simulink model "c00007M_harness"  (R2018a)
settings: Solver=FixedStepAuto  StartTime=0.0  StopTime=300  FixedStep=0.1  RelTol=1e-3
undefined symbols (not defined in the file): A1, hmax, R1, R2, sigbuilder_block, TempThreshold
(part 4 of 14)

== system c00007M_harness/M014/Tank1 ==
  CT1 : Inport
  F1 : Inport  Port=2
  E1 : Inport  Port=3
  MR1 : Inport  Port=4
  T1 : Inport  Port=5
  EB1 : Inport  Port=6
  Control : Subsystem
  Memory : Memory
  TankModel : Subsystem
  LL1 : Outport
  wires:
  TankModel/1(LiquidLevel) -> Memory/1, LL1/1
  Control/2(LiquidOut) -> TankModel/2(LiquidOut)
  Memory/1 -> Control/8(LiquidLevel)
  MR1/1 -> Control/3(ManualReference)
  CT1/1 -> Control/2(StartMaintenance), Control/1(ControlType)
  F1/1 -> Control/4(Fill)
  E1/1 -> Control/5(Empty)
  EB1/1 -> Control/6(EmergencyButton)
  T1/1 -> Control/7(Temperature)
  Control/1(LiquidIn) -> TankModel/1(LiquidIn)

== system c00007M_harness/M015/Tank1 ==
  CT1 : Inport
  F1 : Inport  Port=2
  E1 : Inport  Port=3
  MR1 : Inport  Port=4
  T1 : Inport  Port=5
  EB1 : Inport  Port=6
  Control : Subsystem
  Memory : Memory
  TankModel : Subsystem
  LL1 : Outport
  wires:
  TankModel/1(LiquidLevel) -> Memory/1, LL1/1
  Control/2(LiquidOut) -> TankModel/2(LiquidOut)
  Memory/1 -> Control/8(LiquidLevel)
  MR1/1 -> Control/3(ManualReference)
  CT1/1 -> Control/2(StartMaintenance), Control/1(ControlType)
  F1/1 -> Control/4(Fill)
  E1/1 -> Control/5(Empty)
  EB1/1 -> Control/6(EmergencyButton)
  T1/1 -> Control/7(Temperature)
  Control/1(LiquidIn) -> TankModel/1(LiquidIn)

== system c00007M_harness/M016/Tank1 ==
  CT1 : Inport
  F1 : Inport  Port=2
  E1 : Inport  Port=3
  MR1 : Inport  Port=4
  T1 : Inport  Port=5
  EB1 : Inport  Port=6
  Control : Subsystem
  Memory : Memory
  TankModel : Subsystem
  LL1 : Outport
  wires:
  TankModel/1(LiquidLevel) -> Memory/1, LL1/1
  Control/2(LiquidOut) -> TankModel/2(LiquidOut)
  Memory/1 -> Control/8(LiquidLevel)
  MR1/1 -> Control/3(ManualReference)
  CT1/1 -> Control/2(StartMaintenance), Control/1(ControlType)
  F1/1 -> Control/4(Fill)
  E1/1 -> Control/5(Empty)
  EB1/1 -> Control/6(EmergencyButton)
  T1/1 -> Control/7(Temperature)
  Control/1(LiquidIn) -> TankModel/1(LiquidIn)

== system c00007M_harness/M017/Tank1 ==
  CT1 : Inport
  F1 : Inport  Port=2
  E1 : Inport  Port=3
  MR1 : Inport  Port=4
  T1 : Inport  Port=5
  EB1 : Inport  Port=6
  Control : Subsystem
  Memory : Memory
  TankModel : Subsystem
  LL1 : Outport
  wires:
  TankModel/1(LiquidLevel) -> Memory/1, LL1/1
  Control/2(LiquidOut) -> TankModel/2(LiquidOut)
  Memory/1 -> Control/8(LiquidLevel)
  MR1/1 -> Control/3(ManualReference)
  CT1/1 -> Control/2(StartMaintenance), Control/1(ControlType)
  F1/1 -> Control/4(Fill)
  E1/1 -> Control/5(Empty)
  EB1/1 -> Control/6(EmergencyButton)
  T1/1 -> Control/7(Temperature)
  Control/1(LiquidIn) -> TankModel/1(LiquidIn)

== system c00007M_harness/M018/Tank1 ==
  CT1 : Inport
  F1 : Inport  Port=2
  E1 : Inport  Port=3
  MR1 : Inport  Port=4
  T1 : Inport  Port=5
  EB1 : Inport  Port=6
  Control : Subsystem
  Memory : Memory
  TankModel : Subsystem
  LL1 : Outport
  wires:
  TankModel/1(LiquidLevel) -> Memory/1, LL1/1
  Control/2(LiquidOut) -> TankModel/2(LiquidOut)
  Memory/1 -> Control/8(LiquidLevel)
  MR1/1 -> Control/3(ManualReference)
  CT1/1 -> Control/2(StartMaintenance), Control/1(ControlType)
  F1/1 -> Control/4(Fill)
  E1/1 -> Control/5(Empty)
  EB1/1 -> Control/6(EmergencyButton)
  T1/1 -> Control/7(Temperature)
  Control/1(LiquidIn) -> TankModel/1(LiquidIn)

== system c00007M_harness/M019/Tank1 ==
  CT1 : Inport
  F1 : Inport  Port=2
  E1 : Inport  Port=3
  MR1 : Inport  Port=4
  T1 : Inport  Port=5
  EB1 : Inport  Port=6
  Control : Subsystem
  Memory : Memory
  TankModel : Subsystem
  LL1 : Outport
  wires:
  TankModel/1(LiquidLevel) -> Memory/1, LL1/1
  Control/2(LiquidOut) -> TankModel/2(LiquidOut)
  Memory/1 -> Control/8(LiquidLevel)
  MR1/1 -> Control/3(ManualReference)
  CT1/1 -> Control/2(StartMaintenance), Control/1(ControlType)
  F1/1 -> Control/4(Fill)
  E1/1 -> Control/5(Empty)
  EB1/1 -> Control/6(EmergencyButton)
  T1/1 -> Control/7(Temperature)
  Control/1(LiquidIn) -> TankModel/1(LiquidIn)

== system c00007M_harness/M020/Tank1 ==
  CT1 : Inport
  F1 : Inport  Port=2
  E1 : Inport  Port=3
  MR1 : Inport  Port=4
  T1 : Inport  Port=5
  EB1 : Inport  Port=6
  Control : Subsystem
  Memory : Memory
  TankModel : Subsystem
  LL1 : Outport
  wires:
  TankModel/1(LiquidLevel) -> Memory/1, LL1/1
  Control/2(LiquidOut) -> TankModel/2(LiquidOut)
  Memory/1 -> Control/8(LiquidLevel)
  MR1/1 -> Control/3(ManualReference)
  CT1/1 -> Control/2(StartMaintenance), Control/1(ControlType)
  F1/1 -> Control/4(Fill)
  E1/1 -> Control/5(Empty)
  EB1/1 -> Control/6(EmergencyButton)
  T1/1 -> Control/7(Temperature)
  Control/1(LiquidIn) -> TankModel/1(LiquidIn)

== system c00007M_harness/M021/Tank1 ==
  CT1 : Inport
  F1 : Inport  Port=2
  E1 : Inport  Port=3
  MR1 : Inport  Port=4
  T1 : Inport  Port=5
  EB1 : Inport  Port=6
  Control : Subsystem
  Memory : Memory
  TankModel : Subsystem
  LL1 : Outport
  wires:
  TankModel/1(LiquidLevel) -> Memory/1, LL1/1
  Control/2(LiquidOut) -> TankModel/2(LiquidOut)
  Memory/1 -> Control/8(LiquidLevel)
  MR1/1 -> Control/3(ManualReference)
  CT1/1 -> Control/2(StartMaintenance), Control/1(ControlType)
  F1/1 -> Control/4(Fill)
  E1/1 -> Control/5(Empty)
  EB1/1 -> Control/6(EmergencyButton)
  T1/1 -> Control/7(Temperature)
  Control/1(LiquidIn) -> TankModel/1(LiquidIn)

== system c00007M_harness/M022/Tank1 ==
  CT1 : Inport
  F1 : Inport  Port=2
  E1 : Inport  Port=3
  MR1 : Inport  Port=4
  T1 : Inport  Port=5
  EB1 : Inport  Port=6
  Control : Subsystem
  Memory : Memory
  TankModel : Subsystem
  LL1 : Outport
  wires:
  TankModel/1(LiquidLevel) -> Memory/1, LL1/1
  Control/2(LiquidOut) -> TankModel/2(LiquidOut)
  Memory/1 -> Control/8(LiquidLevel)
  MR1/1 -> Control/3(ManualReference)
  CT1/1 -> Control/2(StartMaintenance), Control/1(ControlType)
  F1/1 -> Control/4(Fill)
  E1/1 -> Control/5(Empty)
  EB1/1 -> Control/6(EmergencyButton)
  T1/1 -> Control/7(Temperature)
  Control/1(LiquidIn) -> TankModel/1(LiquidIn)

== system c00007M_harness/M023/Tank1 ==
  CT1 : Inport
  F1 : Inport  Port=2
  E1 : Inport  Port=3
  MR1 : Inport  Port=4
  T1 : Inport  Port=5
  EB1 : Inport  Port=6
  Control : Subsystem
  Memory : Memory
  TankModel : Subsystem
  LL1 : Outport
  wires:
  TankModel/1(LiquidLevel) -> Memory/1, LL1/1
  Control/2(LiquidOut) -> TankModel/2(LiquidOut)
  Memory/1 -> Control/8(LiquidLevel)
  MR1/1 -> Control/3(ManualReference)
  CT1/1 -> Control/2(StartMaintenance), Control/1(ControlType)
  F1/1 -> Control/4(Fill)
  E1/1 -> Control/5(Empty)
  EB1/1 -> Control/6(EmergencyButton)
  T1/1 -> Control/7(Temperature)
  Control/1(LiquidIn) -> TankModel/1(LiquidIn)

== system c00007M_harness/M024/Tank1 ==
  CT1 : Inport
  F1 : Inport  Port=2
  E1 : Inport  Port=3
  MR1 : Inport  Port=4
  T1 : Inport  Port=5
  EB1 : Inport  Port=6
  Control : Subsystem
  Memory : Memory
  TankModel : Subsystem
  LL1 : Outport
  wires:
  TankModel/1(LiquidLevel) -> Memory/1, LL1/1
  Control/2(LiquidOut) -> TankModel/2(LiquidOut)
  Memory/1 -> Control/8(LiquidLevel)
  MR1/1 -> Control/3(ManualReference)
  CT1/1 -> Control/2(StartMaintenance), Control/1(ControlType)
  F1/1 -> Control/4(Fill)
  E1/1 -> Control/5(Empty)
  EB1/1 -> Control/6(EmergencyButton)
  T1/1 -> Control/7(Temperature)
  Control/1(LiquidIn) -> TankModel/1(LiquidIn)

== system c00007M_harness/M025/Tank1 ==
  CT1 : Inport
  F1 : Inport  Port=2
  E1 : Inport  Port=3
  MR1 : Inport  Port=4
  T1 : Inport  Port=5
  EB1 : Inport  Port=6
  Control : Subsystem
  Memory : Memory
  TankModel : Subsystem
  LL1 : Outport
  wires:
  TankModel/1(LiquidLevel) -> Memory/1, LL1/1
  Control/2(LiquidOut) -> TankModel/2(LiquidOut)
  Memory/1 -> Control/8(LiquidLevel)
  MR1/1 -> Control/3(ManualReference)
  CT1/1 -> Control/2(StartMaintenance), Control/1(ControlType)
  F1/1 -> Control/4(Fill)
  E1/1 -> Control/5(Empty)
  EB1/1 -> Control/6(EmergencyButton)
  T1/1 -> Control/7(Temperature)
  Control/1(LiquidIn) -> TankModel/1(LiquidIn)

== system c00007M_harness/M026/Tank1 ==
  CT1 : Inport
  F1 : Inport  Port=2
  E1 : Inport  Port=3
  MR1 : Inport  Port=4
  T1 : Inport  Port=5
  EB1 : Inport  Port=6
  Control : Subsystem
  Memory : Memory
  TankModel : Subsystem
  LL1 : Outport
  wires:
  TankModel/1(LiquidLevel) -> Memory/1, LL1/1
  Control/2(LiquidOut) -> TankModel/2(LiquidOut)
  Memory/1 -> Control/8(LiquidLevel)
  MR1/1 -> Control/3(ManualReference)
  CT1/1 -> Control/2(StartMaintenance), Control/1(ControlType)
  F1/1 -> Control/4(Fill)
  E1/1 -> Control/5(Empty)
  EB1/1 -> Control/6(EmergencyButton)
  T1/1 -> Control/7(Temperature)
  Control/1(LiquidIn) -> TankModel/1(LiquidIn)

== system c00007M_harness/M027/Tank1 ==
  CT1 : Inport
  F1 : Inport  Port=2
  E1 : Inport  Port=3
  MR1 : Inport  Port=4
  T1 : Inport  Port=5
  EB1 : Inport  Port=6
  Control : Subsystem
  Memory : Memory
  TankModel : Subsystem
  LL1 : Outport
  wires:
  TankModel/1(LiquidLevel) -> Memory/1, LL1/1
  Control/2(LiquidOut) -> TankModel/2(LiquidOut)
  Memory/1 -> Control/8(LiquidLevel)
  MR1/1 -> Control/3(ManualReference)
  CT1/1 -> Control/2(StartMaintenance), Control/1(ControlType)
  F1/1 -> Control/4(Fill)
  E1/1 -> Control/5(Empty)
  EB1/1 -> Control/6(EmergencyButton)
  T1/1 -> Control/7(Temperature)
  Control/1(LiquidIn) -> TankModel/1(LiquidIn)

== system c00007M_harness/M028/Tank1 ==
  CT1 : Inport
  F1 : Inport  Port=2
  E1 : Inport  Port=3
  MR1 : Inport  Port=4
  T1 : Inport  Port=5
  EB1 : Inport  Port=6
  Control : Subsystem
  Memory : Memory
  TankModel : Subsystem
  LL1 : Outport
  wires:
  TankModel/1(LiquidLevel) -> Memory/1, LL1/1
  Control/2(LiquidOut) -> TankModel/2(LiquidOut)
  Memory/1 -> Control/8(LiquidLevel)
  MR1/1 -> Control/3(ManualReference)
  CT1/1 -> Control/2(StartMaintenance), Control/1(ControlType)
  F1/1 -> Control/4(Fill)
  E1/1 -> Control/5(Empty)
  EB1/1 -> Control/6(EmergencyButton)
  T1/1 -> Control/7(Temperature)
  Control/1(LiquidIn) -> TankModel/1(LiquidIn)

== system c00007M_harness/M029/Tank1 ==
  CT1 : Inport
  F1 : Inport  Port=2
  E1 : Inport  Port=3
  MR1 : Inport  Port=4
  T1 : Inport  Port=5
  EB1 : Inport  Port=6
  Control : Subsystem
  Memory : Memory
  TankModel : Subsystem
  LL1 : Outport
  wires:
  TankModel/1(LiquidLevel) -> Memory/1, LL1/1
  Control/2(LiquidOut) -> TankModel/2(LiquidOut)
  Memory/1 -> Control/8(LiquidLevel)
  MR1/1 -> Control/3(ManualReference)
  CT1/1 -> Control/2(StartMaintenance), Control/1(ControlType)
  F1/1 -> Control/4(Fill)
  E1/1 -> Control/5(Empty)
  EB1/1 -> Control/6(EmergencyButton)
  T1/1 -> Control/7(Temperature)
  Control/1(LiquidIn) -> TankModel/1(LiquidIn)

== system c00007M_harness/M030/Tank1 ==
  CT1 : Inport
  F1 : Inport  Port=2
  E1 : Inport  Port=3
  MR1 : Inport  Port=4
  T1 : Inport  Port=5
  EB1 : Inport  Port=6
  Control : Subsystem
  Memory : Memory
  TankModel : Subsystem
  LL1 : Outport
  wires:
  TankModel/1(LiquidLevel) -> Memory/1, LL1/1
  Control/2(LiquidOut) -> TankModel/2(LiquidOut)
  Memory/1 -> Control/8(LiquidLevel)
  MR1/1 -> Control/3(ManualReference)
  CT1/1 -> Control/2(StartMaintenance), Control/1(ControlType)
  F1/1 -> Control/4(Fill)
  E1/1 -> Control/5(Empty)
  EB1/1 -> Control/6(EmergencyButton)
  T1/1 -> Control/7(Temperature)
  Control/1(LiquidIn) -> TankModel/1(LiquidIn)

== system c00007M_harness/M031/Tank1 ==
  CT1 : Inport
  F1 : Inport  Port=2
  E1 : Inport  Port=3
  MR1 : Inport  Port=4
  T1 : Inport  Port=5
  EB1 : Inport  Port=6
  Control : Subsystem
  Memory : Memory
  TankModel : Subsystem
  LL1 : Outport
  wires:
  TankModel/1(LiquidLevel) -> Memory/1, LL1/1
  Control/2(LiquidOut) -> TankModel/2(LiquidOut)
  Memory/1 -> Control/8(LiquidLevel)
  MR1/1 -> Control/3(ManualReference)
  CT1/1 -> Control/2(StartMaintenance), Control/1(ControlType)
  F1/1 -> Control/4(Fill)
  E1/1 -> Control/5(Empty)
  EB1/1 -> Control/6(EmergencyButton)
  T1/1 -> Control/7(Temperature)
  Control/1(LiquidIn) -> TankModel/1(LiquidIn)

== system c00007M_harness/M032/Tank1 ==
  CT1 : Inport
  F1 : Inport  Port=2
  E1 : Inport  Port=3
  MR1 : Inport  Port=4
  T1 : Inport  Port=5
  EB1 : Inport  Port=6
  Control : Subsystem
  Memory : Memory
  TankModel : Subsystem
  LL1 : Outport
  wires:
  TankModel/1(LiquidLevel) -> Memory/1, LL1/1
  Control/2(LiquidOut) -> TankModel/2(LiquidOut)
  Memory/1 -> Control/8(LiquidLevel)
  MR1/1 -> Control/3(ManualReference)
  CT1/1 -> Control/2(StartMaintenance), Control/1(ControlType)
  F1/1 -> Control/4(Fill)
  E1/1 -> Control/5(Empty)
  EB1/1 -> Control/6(EmergencyButton)
  T1/1 -> Control/7(Temperature)
  Control/1(LiquidIn) -> TankModel/1(LiquidIn)

== system c00007M_harness/M033/Tank1 ==
  CT1 : Inport
  F1 : Inport  Port=2
  E1 : Inport  Port=3
  MR1 : Inport  Port=4
  T1 : Inport  Port=5
  EB1 : Inport  Port=6
  Control : Subsystem
  Memory : Memory
  TankModel : Subsystem
  LL1 : Outport
  wires:
  TankModel/1(LiquidLevel) -> Memory/1, LL1/1
  Control/2(LiquidOut) -> TankModel/2(LiquidOut)
  Memory/1 -> Control/8(LiquidLevel)
  MR1/1 -> Control/3(ManualReference)
  CT1/1 -> Control/2(StartMaintenance), Control/1(ControlType)
  F1/1 -> Control/4(Fill)
  E1/1 -> Control/5(Empty)
  EB1/1 -> Control/6(EmergencyButton)
  T1/1 -> Control/7(Temperature)
  Control/1(LiquidIn) -> TankModel/1(LiquidIn)

== system c00007M_harness/M034/Tank1 ==
  CT1 : Inport
  F1 : Inport  Port=2
  E1 : Inport  Port=3
  MR1 : Inport  Port=4
  T1 : Inport  Port=5
  EB1 : Inport  Port=6
  Control : Subsystem
  Memory : Memory
  TankModel : Subsystem
  LL1 : Outport
  wires:
  TankModel/1(LiquidLevel) -> Memory/1, LL1/1
  Control/2(LiquidOut) -> TankModel/2(LiquidOut)
  Memory/1 -> Control/8(LiquidLevel)
  MR1/1 -> Control/3(ManualReference)
  CT1/1 -> Control/2(StartMaintenance), Control/1(ControlType)
  F1/1 -> Control/4(Fill)
  E1/1 -> Control/5(Empty)
  EB1/1 -> Control/6(EmergencyButton)
  T1/1 -> Control/7(Temperature)
  Control/1(LiquidIn) -> TankModel/1(LiquidIn)

== system c00007M_harness/M035/Tank1 ==
  CT1 : Inport
  F1 : Inport  Port=2
  E1 : Inport  Port=3
  MR1 : Inport  Port=4
  T1 : Inport  Port=5
  EB1 : Inport  Port=6
  Control : Subsystem
  Memory : Memory
  TankModel : Subsystem
  LL1 : Outport
  wires:
  TankModel/1(LiquidLevel) -> Memory/1, LL1/1
  Control/2(LiquidOut) -> TankModel/2(LiquidOut)
  Memory/1 -> Control/8(LiquidLevel)
  MR1/1 -> Control/3(ManualReference)
  CT1/1 -> Control/2(StartMaintenance), Control/1(ControlType)
  F1/1 -> Control/4(Fill)
  E1/1 -> Control/5(Empty)
  EB1/1 -> Control/6(EmergencyButton)
  T1/1 -> Control/7(Temperature)
  Control/1(LiquidIn) -> TankModel/1(LiquidIn)

== system c00007M_harness/M036/Tank1 ==
  CT1 : Inport
  F1 : Inport  Port=2
  E1 : Inport  Port=3
  MR1 : Inport  Port=4
  T1 : Inport  Port=5
  EB1 : Inport  Port=6
  Control : Subsystem
  Memory : Memory
  TankModel : Subsystem
  LL1 : Outport
  wires:
  TankModel/1(LiquidLevel) -> Memory/1, LL1/1
  Control/2(LiquidOut) -> TankModel/2(LiquidOut)
  Memory/1 -> Control/8(LiquidLevel)
  MR1/1 -> Control/3(ManualReference)
  CT1/1 -> Control/2(StartMaintenance), Control/1(ControlType)
  F1/1 -> Control/4(Fill)
  E1/1 -> Control/5(Empty)
  EB1/1 -> Control/6(EmergencyButton)
  T1/1 -> Control/7(Temperature)
  Control/1(LiquidIn) -> TankModel/1(LiquidIn)

== system c00007M_harness/M037/Tank1 ==
  CT1 : Inport
  F1 : Inport  Port=2
  E1 : Inport  Port=3
  MR1 : Inport  Port=4
  T1 : Inport  Port=5
  EB1 : Inport  Port=6
  Control : Subsystem
  Memory : Memory
  TankModel : Subsystem
  LL1 : Outport
  wires:
  TankModel/1(LiquidLevel) -> Memory/1, LL1/1
  Control/2(LiquidOut) -> TankModel/2(LiquidOut)
  Memory/1 -> Control/8(LiquidLevel)
  MR1/1 -> Control/3(ManualReference)
  CT1/1 -> Control/2(StartMaintenance), Control/1(ControlType)
  F1/1 -> Control/4(Fill)
  E1/1 -> Control/5(Empty)
  EB1/1 -> Control/6(EmergencyButton)
  T1/1 -> Control/7(Temperature)
  Control/1(LiquidIn) -> TankModel/1(LiquidIn)

== system c00007M_harness/M038/Tank1 ==
  CT1 : Inport
  F1 : Inport  Port=2
  E1 : Inport  Port=3
  MR1 : Inport  Port=4
  T1 : Inport  Port=5
  EB1 : Inport  Port=6
  Control : Subsystem
  Memory : Memory
  TankModel : Subsystem
  LL1 : Outport
  wires:
  TankModel/1(LiquidLevel) -> Memory/1, LL1/1
  Control/2(LiquidOut) -> TankModel/2(LiquidOut)
  Memory/1 -> Control/8(LiquidLevel)
  MR1/1 -> Control/3(ManualReference)
  CT1/1 -> Control/2(StartMaintenance), Control/1(ControlType)
  F1/1 -> Control/4(Fill)
  E1/1 -> Control/5(Empty)
  EB1/1 -> Control/6(EmergencyButton)
  T1/1 -> Control/7(Temperature)
  Control/1(LiquidIn) -> TankModel/1(LiquidIn)

== system c00007M_harness/M039/Tank1 ==
  CT1 : Inport
  F1 : Inport  Port=2
  E1 : Inport  Port=3
  MR1 : Inport  Port=4
  T1 : Inport  Port=5
  EB1 : Inport  Port=6
  Control : Subsystem
  Memory : Memory
  TankModel : Subsystem
  LL1 : Outport
  wires:
  TankModel/1(LiquidLevel) -> Memory/1, LL1/1
  Control/2(LiquidOut) -> TankModel/2(LiquidOut)
  Memory/1 -> Control/8(LiquidLevel)
  MR1/1 -> Control/3(ManualReference)
  CT1/1 -> Control/2(StartMaintenance), Control/1(ControlType)
  F1/1 -> Control/4(Fill)
  E1/1 -> Control/5(Empty)
  EB1/1 -> Control/6(EmergencyButton)
  T1/1 -> Control/7(Temperature)
  Control/1(LiquidIn) -> TankModel/1(LiquidIn)

== system c00007M_harness/M040/Tank1 ==
  CT1 : Inport
  F1 : Inport  Port=2
  E1 : Inport  Port=3
  MR1 : Inport  Port=4
  T1 : Inport  Port=5
  EB1 : Inport  Port=6
  Control : Subsystem
  Memory : Memory
  TankModel : Subsystem
  LL1 : Outport
  wires:
  TankModel/1(LiquidLevel) -> Memory/1, LL1/1
  Control/2(LiquidOut) -> TankModel/2(LiquidOut)
  Memory/1 -> Control/8(LiquidLevel)
  MR1/1 -> Control/3(ManualReference)
  CT1/1 -> Control/2(StartMaintenance), Control/1(ControlType)
  F1/1 -> Control/4(Fill)
  E1/1 -> Control/5(Empty)
  EB1/1 -> Control/6(EmergencyButton)
  T1/1 -> Control/7(Temperature)
  Control/1(LiquidIn) -> TankModel/1(LiquidIn)

== system c00007M_harness/M041/Tank1 ==
  CT1 : Inport
  F1 : Inport  Port=2
  E1 : Inport  Port=3
  MR1 : Inport  Port=4
  T1 : Inport  Port=5
  EB1 : Inport  Port=6
  Control : Subsystem
  Memory : Memory
  TankModel : Subsystem
  LL1 : Outport
  wires:
  TankModel/1(LiquidLevel) -> Memory/1, LL1/1
  Control/2(LiquidOut) -> TankModel/2(LiquidOut)
  Memory/1 -> Control/8(LiquidLevel)
  MR1/1 -> Control/3(ManualReference)
  CT1/1 -> Control/2(StartMaintenance), Control/1(ControlType)
  F1/1 -> Control/4(Fill)
  E1/1 -> Control/5(Empty)
  EB1/1 -> Control/6(EmergencyButton)
  T1/1 -> Control/7(Temperature)
  Control/1(LiquidIn) -> TankModel/1(LiquidIn)

== system c00007M_harness/M042/Tank1 ==
  CT1 : Inport
  F1 : Inport  Port=2
  E1 : Inport  Port=3
  MR1 : Inport  Port=4
  T1 : Inport  Port=5
  EB1 : Inport  Port=6
  Control : Subsystem
  Memory : Memory
  TankModel : Subsystem
  LL1 : Outport
  wires:
  TankModel/1(LiquidLevel) -> Memory/1, LL1/1
  Control/2(LiquidOut) -> TankModel/2(LiquidOut)
  Memory/1 -> Control/8(LiquidLevel)
  MR1/1 -> Control/3(ManualReference)
  CT1/1 -> Control/2(StartMaintenance), Control/1(ControlType)
  F1/1 -> Control/4(Fill)
  E1/1 -> Control/5(Empty)
  EB1/1 -> Control/6(EmergencyButton)
  T1/1 -> Control/7(Temperature)
  Control/1(LiquidIn) -> TankModel/1(LiquidIn)

== system c00007M_harness/M043/Tank1 ==
  CT1 : Inport
  F1 : Inport  Port=2
  E1 : Inport  Port=3
  MR1 : Inport  Port=4
  T1 : Inport  Port=5
  EB1 : Inport  Port=6
  Control : Subsystem
  Memory : Memory
  TankModel : Subsystem
  LL1 : Outport
  wires:
  TankModel/1(LiquidLevel) -> Memory/1, LL1/1
  Control/2(LiquidOut) -> TankModel/2(LiquidOut)
  Memory/1 -> Control/8(LiquidLevel)
  MR1/1 -> Control/3(ManualReference)
  CT1/1 -> Control/2(StartMaintenance), Control/1(ControlType)
  F1/1 -> Control/4(Fill)
  E1/1 -> Control/5(Empty)
  EB1/1 -> Control/6(EmergencyButton)
  T1/1 -> Control/7(Temperature)
  Control/1(LiquidIn) -> TankModel/1(LiquidIn)

== system c00007M_harness/M044/Tank1 ==
  CT1 : Inport
  F1 : Inport  Port=2
  E1 : Inport  Port=3
  MR1 : Inport  Port=4
  T1 : Inport  Port=5
  EB1 : Inport  Port=6
  Control : Subsystem
  Memory : Memory
  TankModel : Subsystem
  LL1 : Outport
  wires:
  TankModel/1(LiquidLevel) -> Memory/1, LL1/1
  Control/2(LiquidOut) -> TankModel/2(LiquidOut)
  Memory/1 -> Control/8(LiquidLevel)
  MR1/1 -> Control/3(ManualReference)
  CT1/1 -> Control/2(StartMaintenance), Control/1(ControlType)
  F1/1 -> Control/4(Fill)
  E1/1 -> Control/5(Empty)
  EB1/1 -> Control/6(EmergencyButton)
  T1/1 -> Control/7(Temperature)
  Control/1(LiquidIn) -> TankModel/1(LiquidIn)

== system c00007M_harness/M045/Tank1 ==
  CT1 : Inport
  F1 : Inport  Port=2
  E1 : Inport  Port=3
  MR1 : Inport  Port=4
  T1 : Inport  Port=5
  EB1 : Inport  Port=6
  Control : Subsystem
  Memory : Memory
  TankModel : Subsystem
  LL1 : Outport
  wires:
  TankModel/1(LiquidLevel) -> Memory/1, LL1/1
  Control/2(LiquidOut) -> TankModel/2(LiquidOut)
  Memory/1 -> Control/8(LiquidLevel)
  MR1/1 -> Control/3(ManualReference)
  CT1/1 -> Control/2(StartMaintenance), Control/1(ControlType)
  F1/1 -> Control/4(Fill)
  E1/1 -> Control/5(Empty)
  EB1/1 -> Control/6(EmergencyButton)
  T1/1 -> Control/7(Temperature)
  Control/1(LiquidIn) -> TankModel/1(LiquidIn)

== system c00007M_harness/M046/Tank1 ==
  CT1 : Inport
  F1 : Inport  Port=2
  E1 : Inport  Port=3
  MR1 : Inport  Port=4
  T1 : Inport  Port=5
  EB1 : Inport  Port=6
  Control : Subsystem
  Memory : Memory
  TankModel : Subsystem
  LL1 : Outport
  wires:
  TankModel/1(LiquidLevel) -> Memory/1, LL1/1
  Control/2(LiquidOut) -> TankModel/2(LiquidOut)
  Memory/1 -> Control/8(LiquidLevel)
  MR1/1 -> Control/3(ManualReference)
  CT1/1 -> Control/2(StartMaintenance), Control/1(ControlType)
  F1/1 -> Control/4(Fill)
  E1/1 -> Control/5(Empty)
  EB1/1 -> Control/6(EmergencyButton)
  T1/1 -> Control/7(Temperature)
  Control/1(LiquidIn) -> TankModel/1(LiquidIn)

== system c00007M_harness/M047/Tank1 ==
  CT1 : Inport
  F1 : Inport  Port=2
  E1 : Inport  Port=3
  MR1 : Inport  Port=4
  T1 : Inport  Port=5
  EB1 : Inport  Port=6
  Control : Subsystem
  Memory : Memory
  TankModel : Subsystem
  LL1 : Outport
  wires:
  TankModel/1(LiquidLevel) -> Memory/1, LL1/1
  Control/2(LiquidOut) -> TankModel/2(LiquidOut)
  Memory/1 -> Control/8(LiquidLevel)
  MR1/1 -> Control/3(ManualReference)
  CT1/1 -> Control/2(StartMaintenance), Control/1(ControlType)
  F1/1 -> Control/4(Fill)
  E1/1 -> Control/5(Empty)
  EB1/1 -> Control/6(EmergencyButton)
  T1/1 -> Control/7(Temperature)
  Control/1(LiquidIn) -> TankModel/1(LiquidIn)

== system c00007M_harness/M048/Tank1 ==
  CT1 : Inport
  F1 : Inport  Port=2
  E1 : Inport  Port=3
  MR1 : Inport  Port=4
  T1 : Inport  Port=5
  EB1 : Inport  Port=6
  Control : Subsystem
  Memory : Memory
  TankModel : Subsystem
  LL1 : Outport
  wires:
  TankModel/1(LiquidLevel) -> Memory/1, LL1/1
  Control/2(LiquidOut) -> TankModel/2(LiquidOut)
  Memory/1 -> Control/8(LiquidLevel)
  MR1/1 -> Control/3(ManualReference)
  CT1/1 -> Control/2(StartMaintenance), Control/1(ControlType)
  F1/1 -> Control/4(Fill)
  E1/1 -> Control/5(Empty)
  EB1/1 -> Control/6(EmergencyButton)
  T1/1 -> Control/7(Temperature)
  Control/1(LiquidIn) -> TankModel/1(LiquidIn)

== system c00007M_harness/M049/Tank1 ==
  CT1 : Inport
  F1 : Inport  Port=2
  E1 : Inport  Port=3
  MR1 : Inport  Port=4
  T1 : Inport  Port=5
  EB1 : Inport  Port=6
  Control : Subsystem
  Memory : Memory
  TankModel : Subsystem
  LL1 : Outport
  wires:
  TankModel/1(LiquidLevel) -> Memory/1, LL1/1
  Control/2(LiquidOut) -> TankModel/2(LiquidOut)
  Memory/1 -> Control/8(LiquidLevel)
  MR1/1 -> Control/3(ManualReference)
  CT1/1 -> Control/2(StartMaintenance), Control/1(ControlType)
  F1/1 -> Control/4(Fill)
  E1/1 -> Control/5(Empty)
  EB1/1 -> Control/6(EmergencyButton)
  T1/1 -> Control/7(Temperature)
  Control/1(LiquidIn) -> TankModel/1(LiquidIn)

== system c00007M_harness/M050/Tank1 ==
  CT1 : Inport
  F1 : Inport  Port=2
  E1 : Inport  Port=3
  MR1 : Inport  Port=4
  T1 : Inport  Port=5
  EB1 : Inport  Port=6
  Control : Subsystem
  Memory : Memory
  TankModel : Subsystem
  LL1 : Outport
  wires:
  TankModel/1(LiquidLevel) -> Memory/1, LL1/1
  Control/2(LiquidOut) -> TankModel/2(LiquidOut)
  Memory/1 -> Control/8(LiquidLevel)
  MR1/1 -> Control/3(ManualReference)
  CT1/1 -> Control/2(StartMaintenance), Control/1(ControlType)
  F1/1 -> Control/4(Fill)
  E1/1 -> Control/5(Empty)
  EB1/1 -> Control/6(EmergencyButton)
  T1/1 -> Control/7(Temperature)
  Control/1(LiquidIn) -> TankModel/1(LiquidIn)

== system c00007M_harness/M051/Tank1 ==
  CT1 : Inport
  F1 : Inport  Port=2
  E1 : Inport  Port=3
  MR1 : Inport  Port=4
  T1 : Inport  Port=5
  EB1 : Inport  Port=6
  Control : Subsystem
  Memory : Memory
  TankModel : Subsystem
  LL1 : Outport
  wires:
  TankModel/1(LiquidLevel) -> Memory/1, LL1/1
  Control/2(LiquidOut) -> TankModel/2(LiquidOut)
  Memory/1 -> Control/8(LiquidLevel)
  MR1/1 -> Control/3(ManualReference)
  CT1/1 -> Control/2(StartMaintenance), Control/1(ControlType)
  F1/1 -> Control/4(Fill)
  E1/1 -> Control/5(Empty)
  EB1/1 -> Control/6(EmergencyButton)
  T1/1 -> Control/7(Temperature)
  Control/1(LiquidIn) -> TankModel/1(LiquidIn)

== system c00007M_harness/M052/Tank1 ==
  CT1 : Inport
  F1 : Inport  Port=2
  E1 : Inport  Port=3
  MR1 : Inport  Port=4
  T1 : Inport  Port=5
  EB1 : Inport  Port=6
  Control : Subsystem
  Memory : Memory
  TankModel : Subsystem
  LL1 : Outport
  wires:
  TankModel/1(LiquidLevel) -> Memory/1, LL1/1
  Control/2(LiquidOut) -> TankModel/2(LiquidOut)
  Memory/1 -> Control/8(LiquidLevel)
  MR1/1 -> Control/3(ManualReference)
  CT1/1 -> Control/2(StartMaintenance), Control/1(ControlType)
  F1/1 -> Control/4(Fill)
  E1/1 -> Control/5(Empty)
  EB1/1 -> Control/6(EmergencyButton)
  T1/1 -> Control/7(Temperature)
  Control/1(LiquidIn) -> TankModel/1(LiquidIn)

== system c00007M_harness/M053/Tank1 ==
  CT1 : Inport
  F1 : Inport  Port=2
  E1 : Inport  Port=3
  MR1 : Inport  Port=4
  T1 : Inport  Port=5
  EB1 : Inport  Port=6
  Control : Subsystem
  Memory : Memory
  TankModel : Subsystem
  LL1 : Outport
  wires:
  TankModel/1(LiquidLevel) -> Memory/1, LL1/1
  Control/2(LiquidOut) -> TankModel/2(LiquidOut)
  Memory/1 -> Control/8(LiquidLevel)
  MR1/1 -> Control/3(ManualReference)
  CT1/1 -> Control/2(StartMaintenance), Control/1(ControlType)
  F1/1 -> Control/4(Fill)
  E1/1 -> Control/5(Empty)
  EB1/1 -> Control/6(EmergencyButton)
  T1/1 -> Control/7(Temperature)
  Control/1(LiquidIn) -> TankModel/1(LiquidIn)

== system c00007M_harness/M054/Tank1 ==
  CT1 : Inport
  F1 : Inport  Port=2
  E1 : Inport  Port=3
  MR1 : Inport  Port=4
  T1 : Inport  Port=5
  EB1 : Inport  Port=6
  Control : Subsystem
  Memory : Memory
  TankModel : Subsystem
  LL1 : Outport
  wires:
  TankModel/1(LiquidLevel) -> Memory/1, LL1/1
  Control/2(LiquidOut) -> TankModel/2(LiquidOut)
  Memory/1 -> Control/8(LiquidLevel)
  MR1/1 -> Control/3(ManualReference)
  CT1/1 -> Control/2(StartMaintenance), Control/1(ControlType)
  F1/1 -> Control/4(Fill)
  E1/1 -> Control/5(Empty)
  EB1/1 -> Control/6(EmergencyButton)
  T1/1 -> Control/7(Temperature)
  Control/1(LiquidIn) -> TankModel/1(LiquidIn)

== system c00007M_harness/M055/Tank1 ==
  CT1 : Inport
  F1 : Inport  Port=2
  E1 : Inport  Port=3
  MR1 : Inport  Port=4
  T1 : Inport  Port=5
  EB1 : Inport  Port=6
  Control : Subsystem
  Memory : Memory
  TankModel : Subsystem
  LL1 : Outport
  wires:
  TankModel/1(LiquidLevel) -> Memory/1, LL1/1
  Control/2(LiquidOut) -> TankModel/2(LiquidOut)
  Memory/1 -> Control/8(LiquidLevel)
  MR1/1 -> Control/3(ManualReference)
  CT1/1 -> Control/2(StartMaintenance), Control/1(ControlType)
  F1/1 -> Control/4(Fill)
  E1/1 -> Control/5(Empty)
  EB1/1 -> Control/6(EmergencyButton)
  T1/1 -> Control/7(Temperature)
  Control/1(LiquidIn) -> TankModel/1(LiquidIn)

== system c00007M_harness/M056/Tank1 ==
  CT1 : Inport
  F1 : Inport  Port=2
  E1 : Inport  Port=3
  MR1 : Inport  Port=4
  T1 : Inport  Port=5
  EB1 : Inport  Port=6
  Control : Subsystem
  Memory : Memory
  TankModel : Subsystem
  LL1 : Outport
  wires:
  TankModel/1(LiquidLevel) -> Memory/1, LL1/1
  Control/2(LiquidOut) -> TankModel/2(LiquidOut)
  Memory/1 -> Control/8(LiquidLevel)
  MR1/1 -> Control/3(ManualReference)
  CT1/1 -> Control/2(StartMaintenance), Control/1(ControlType)
  F1/1 -> Control/4(Fill)
  E1/1 -> Control/5(Empty)
  EB1/1 -> Control/6(EmergencyButton)
  T1/1 -> Control/7(Temperature)
  Control/1(LiquidIn) -> TankModel/1(LiquidIn)

== system c00007M_harness/M057/Tank1 ==
  CT1 : Inport
  F1 : Inport  Port=2
  E1 : Inport  Port=3
  MR1 : Inport  Port=4
  T1 : Inport  Port=5
  EB1 : Inport  Port=6
  Control : Subsystem
  Memory : Memory
  TankModel : Subsystem
  LL1 : Outport
  wires:
  TankModel/1(LiquidLevel) -> Memory/1, LL1/1
  Control/2(LiquidOut) -> TankModel/2(LiquidOut)
  Memory/1 -> Control/8(LiquidLevel)
  MR1/1 -> Control/3(ManualReference)
  CT1/1 -> Control/2(StartMaintenance), Control/1(ControlType)
  F1/1 -> Control/4(Fill)
  E1/1 -> Control/5(Empty)
  EB1/1 -> Control/6(EmergencyButton)
  T1/1 -> Control/7(Temperature)
  Control/1(LiquidIn) -> TankModel/1(LiquidIn)

== system c00007M_harness/M058/Tank1 ==
  CT1 : Inport
  F1 : Inport  Port=2
  E1 : Inport  Port=3
  MR1 : Inport  Port=4
  T1 : Inport  Port=5
  EB1 : Inport  Port=6
  Control : Subsystem
  Memory : Memory
  TankModel : Subsystem
  LL1 : Outport
  wires:
  TankModel/1(LiquidLevel) -> Memory/1, LL1/1
  Control/2(LiquidOut) -> TankModel/2(LiquidOut)
  Memory/1 -> Control/8(LiquidLevel)
  MR1/1 -> Control/3(ManualReference)
  CT1/1 -> Control/2(StartMaintenance), Control/1(ControlType)
  F1/1 -> Control/4(Fill)
  E1/1 -> Control/5(Empty)
  EB1/1 -> Control/6(EmergencyButton)
  T1/1 -> Control/7(Temperature)
  Control/1(LiquidIn) -> TankModel/1(LiquidIn)

== system c00007M_harness/M059/Tank1 ==
  CT1 : Inport
  F1 : Inport  Port=2
  E1 : Inport  Port=3
  MR1 : Inport  Port=4
  T1 : Inport  Port=5
  EB1 : Inport  Port=6
  Control : Subsystem
  Memory : Memory
  TankModel : Subsystem
  LL1 : Outport
  wires:
  TankModel/1(LiquidLevel) -> Memory/1, LL1/1
  Control/2(LiquidOut) -> TankModel/2(LiquidOut)
  Memory/1 -> Control/8(LiquidLevel)
  MR1/1 -> Control/3(ManualReference)
  CT1/1 -> Control/2(StartMaintenance), Control/1(ControlType)
  F1/1 -> Control/4(Fill)
  E1/1 -> Control/5(Empty)
  EB1/1 -> Control/6(EmergencyButton)
  T1/1 -> Control/7(Temperature)
  Control/1(LiquidIn) -> TankModel/1(LiquidIn)

== system c00007M_harness/M060/Tank1 ==
  CT1 : Inport
  F1 : Inport  Port=2
  E1 : Inport  Port=3
  MR1 : Inport  Port=4
  T1 : Inport  Port=5
  EB1 : Inport  Port=6
  Control : Subsystem
  Memory : Memory
  TankModel : Subsystem
  LL1 : Outport
  wires:
  TankModel/1(LiquidLevel) -> Memory/1, LL1/1
  Control/2(LiquidOut) -> TankModel/2(LiquidOut)
  Memory/1 -> Control/8(LiquidLevel)
  MR1/1 -> Control/3(ManualReference)
  CT1/1 -> Control/2(StartMaintenance), Control/1(ControlType)
  F1/1 -> Control/4(Fill)
  E1/1 -> Control/5(Empty)
  EB1/1 -> Control/6(EmergencyButton)
  T1/1 -> Control/7(Temperature)
  Control/1(LiquidIn) -> TankModel/1(LiquidIn)

== system c00007M_harness/M061/Tank1 ==
  CT1 : Inport
  F1 : Inport  Port=2
  E1 : Inport  Port=3
  MR1 : Inport  Port=4
  T1 : Inport  Port=5
  EB1 : Inport  Port=6
  Control : Subsystem
  Memory : Memory
  TankModel : Subsystem
  LL1 : Outport
  wires:
  TankModel/1(LiquidLevel) -> Memory/1, LL1/1
  Control/2(LiquidOut) -> TankModel/2(LiquidOut)
  Memory/1 -> Control/8(LiquidLevel)
  MR1/1 -> Control/3(ManualReference)
  CT1/1 -> Control/2(StartMaintenance), Control/1(ControlType)
  F1/1 -> Control/4(Fill)
  E1/1 -> Control/5(Empty)
  EB1/1 -> Control/6(EmergencyButton)
  T1/1 -> Control/7(Temperature)
  Control/1(LiquidIn) -> TankModel/1(LiquidIn)

== system c00007M_harness/M069/Tank1 ==
  CT1 : Inport
  F1 : Inport  Port=2
  E1 : Inport  Port=3
  MR1 : Inport  Port=4
  T1 : Inport  Port=5
  EB1 : Inport  Port=6
  Control : Subsystem
  Memory : Memory
  TankModel : Subsystem
  LL1 : Outport
  wires:
  TankModel/1(LiquidLevel) -> Memory/1, LL1/1
  Control/2(LiquidOut) -> TankModel/2(LiquidOut)
  Memory/1 -> Control/8(LiquidLevel)
  MR1/1 -> Control/3(ManualReference)
  CT1/1 -> Control/2(StartMaintenance), Control/1(ControlType)
  F1/1 -> Control/4(Fill)
  E1/1 -> Control/5(Empty)
  EB1/1 -> Control/6(EmergencyButton)
  T1/1 -> Control/7(Temperature)
  Control/1(LiquidIn) -> TankModel/1(LiquidIn)

== system c00007M_harness/M070/Tank1 ==
  CT1 : Inport
  F1 : Inport  Port=2
  E1 : Inport  Port=3
  MR1 : Inport  Port=4
  T1 : Inport  Port=5
  EB1 : Inport  Port=6
  Control : Subsystem
  Memory : Memory
  TankModel : Subsystem
  LL1 : Outport
  wires:
  TankModel/1(LiquidLevel) -> Memory/1, LL1/1
  Control/2(LiquidOut) -> TankModel/2(LiquidOut)
  Memory/1 -> Control/8(LiquidLevel)
  MR1/1 -> Control/3(ManualReference)
  CT1/1 -> Control/2(StartMaintenance), Control/1(ControlType)
  F1/1 -> Control/4(Fill)
  E1/1 -> Control/5(Empty)
  EB1/1 -> Control/6(EmergencyButton)
  T1/1 -> Control/7(Temperature)
  Control/1(LiquidIn) -> TankModel/1(LiquidIn)

== system c00007M_harness/M071/Tank1 ==
  CT1 : Inport
  F1 : Inport  Port=2
  E1 : Inport  Port=3
  MR1 : Inport  Port=4
  T1 : Inport  Port=5
  EB1 : Inport  Port=6
  Control : Subsystem
  Memory : Memory
  TankModel : Subsystem
  LL1 : Outport
  wires:
  TankModel/1(LiquidLevel) -> Memory/1, LL1/1
  Control/2(LiquidOut) -> TankModel/2(LiquidOut)
  Memory/1 -> Control/8(LiquidLevel)
  MR1/1 -> Control/3(ManualReference)
  CT1/1 -> Control/2(StartMaintenance), Control/1(ControlType)
  F1/1 -> Control/4(Fill)
  E1/1 -> Control/5(Empty)
  EB1/1 -> Control/6(EmergencyButton)
  T1/1 -> Control/7(Temperature)
  Control/1(LiquidIn) -> TankModel/1(LiquidIn)

== system c00007M_harness/M072/Tank1 ==
  CT1 : Inport
  F1 : Inport  Port=2
  E1 : Inport  Port=3
  MR1 : Inport  Port=4
  T1 : Inport  Port=5
  EB1 : Inport  Port=6
  Control : Subsystem
  Memory : Memory
  TankModel : Subsystem
  LL1 : Outport
  wires:
  TankModel/1(LiquidLevel) -> Memory/1, LL1/1
  Control/2(LiquidOut) -> TankModel/2(LiquidOut)
  Memory/1 -> Control/8(LiquidLevel)
  MR1/1 -> Control/3(ManualReference)
  CT1/1 -> Control/2(StartMaintenance), Control/1(ControlType)
  F1/1 -> Control/4(Fill)
  E1/1 -> Control/5(Empty)
  EB1/1 -> Control/6(EmergencyButton)
  T1/1 -> Control/7(Temperature)
  Control/1(LiquidIn) -> TankModel/1(LiquidIn)

== system c00007M_harness/M073/Tank1 ==
  CT1 : Inport
  F1 : Inport  Port=2
  E1 : Inport  Port=3
  MR1 : Inport  Port=4
  T1 : Inport  Port=5
  EB1 : Inport  Port=6
  Control : Subsystem
  Memory : Memory
  TankModel : Subsystem
  LL1 : Outport
  wires:
  TankModel/1(LiquidLevel) -> Memory/1, LL1/1
  Control/2(LiquidOut) -> TankModel/2(LiquidOut)
  Memory/1 -> Control/8(LiquidLevel)
  MR1/1 -> Control/3(ManualReference)
  CT1/1 -> Control/2(StartMaintenance), Control/1(ControlType)
  F1/1 -> Control/4(Fill)
  E1/1 -> Control/5(Empty)
  EB1/1 -> Control/6(EmergencyButton)
  T1/1 -> Control/7(Temperature)
  Control/1(LiquidIn) -> TankModel/1(LiquidIn)

== system c00007M_harness/M074/Tank1 ==
  CT1 : Inport
  F1 : Inport  Port=2
  E1 : Inport  Port=3
  MR1 : Inport  Port=4
  T1 : Inport  Port=5
  EB1 : Inport  Port=6
  Control : Subsystem
  Memory : Memory
  TankModel : Subsystem
  LL1 : Outport
  wires:
  TankModel/1(LiquidLevel) -> Memory/1, LL1/1
  Control/2(LiquidOut) -> TankModel/2(LiquidOut)
  Memory/1 -> Control/8(LiquidLevel)
  MR1/1 -> Control/3(ManualReference)
  CT1/1 -> Control/2(StartMaintenance), Control/1(ControlType)
  F1/1 -> Control/4(Fill)
  E1/1 -> Control/5(Empty)
  EB1/1 -> Control/6(EmergencyButton)
  T1/1 -> Control/7(Temperature)
  Control/1(LiquidIn) -> TankModel/1(LiquidIn)

== system c00007M_harness/M075/Tank1 ==
  CT1 : Inport
  F1 : Inport  Port=2
  E1 : Inport  Port=3
  MR1 : Inport  Port=4
  T1 : Inport  Port=5
  EB1 : Inport  Port=6
  Control : Subsystem
  Memory : Memory
  TankModel : Subsystem
  LL1 : Outport
  wires:
  TankModel/1(LiquidLevel) -> Memory/1, LL1/1
  Control/2(LiquidOut) -> TankModel/2(LiquidOut)
  Memory/1 -> Control/8(LiquidLevel)
  MR1/1 -> Control/3(ManualReference)
  CT1/1 -> Control/2(StartMaintenance), Control/1(ControlType)
  F1/1 -> Control/4(Fill)
  E1/1 -> Control/5(Empty)
  EB1/1 -> Control/6(EmergencyButton)
  T1/1 -> Control/7(Temperature)
  Control/1(LiquidIn) -> TankModel/1(LiquidIn)

== system c00007M_harness/M076/Tank1 ==
  CT1 : Inport
  F1 : Inport  Port=2
  E1 : Inport  Port=3
  MR1 : Inport  Port=4
  T1 : Inport  Port=5
  EB1 : Inport  Port=6
  Control : Subsystem
  Memory : Memory
  TankModel : Subsystem
  LL1 : Outport
  wires:
  TankModel/1(LiquidLevel) -> Memory/1, LL1/1
  Control/2(LiquidOut) -> TankModel/2(LiquidOut)
  Memory/1 -> Control/8(LiquidLevel)
  MR1/1 -> Control/3(ManualReference)
  CT1/1 -> Control/2(StartMaintenance), Control/1(ControlType)
  F1/1 -> Control/4(Fill)
  E1/1 -> Control/5(Empty)
  EB1/1 -> Control/6(EmergencyButton)
  T1/1 -> Control/7(Temperature)
  Control/1(LiquidIn) -> TankModel/1(LiquidIn)

== system c00007M_harness/M077/Tank1 ==
  CT1 : Inport
  F1 : Inport  Port=2
  E1 : Inport  Port=3
  MR1 : Inport  Port=4
  T1 : Inport  Port=5
  EB1 : Inport  Port=6
  Control : Subsystem
  Memory : Memory
  TankModel : Subsystem
  LL1 : Outport
  wires:
  TankModel/1(LiquidLevel) -> Memory/1, LL1/1
  Control/2(LiquidOut) -> TankModel/2(LiquidOut)
  Memory/1 -> Control/8(LiquidLevel)
  MR1/1 -> Control/3(ManualReference)
  CT1/1 -> Control/2(StartMaintenance), Control/1(ControlType)
  F1/1 -> Control/4(Fill)
  E1/1 -> Control/5(Empty)
  EB1/1 -> Control/6(EmergencyButton)
  T1/1 -> Control/7(Temperature)
  Control/1(LiquidIn) -> TankModel/1(LiquidIn)

== system c00007M_harness/M078/Tank1 ==
  CT1 : Inport
  F1 : Inport  Port=2
  E1 : Inport  Port=3
  MR1 : Inport  Port=4
  T1 : Inport  Port=5
  EB1 : Inport  Port=6
  Control : Subsystem
  Memory : Memory
  TankModel : Subsystem
  LL1 : Outport
  wires:
  TankModel/1(LiquidLevel) -> Memory/1, LL1/1
  Control/2(LiquidOut) -> TankModel/2(LiquidOut)
  Memory/1 -> Control/8(LiquidLevel)
  MR1/1 -> Control/3(ManualReference)
  CT1/1 -> Control/2(StartMaintenance), Control/1(ControlType)
  F1/1 -> Control/4(Fill)
  E1/1 -> Control/5(Empty)
  EB1/1 -> Control/6(EmergencyButton)
  T1/1 -> Control/7(Temperature)
  Control/1(LiquidIn) -> TankModel/1(LiquidIn)

== system c00007M_harness/M079/Tank1 ==
  CT1 : Inport
  F1 : Inport  Port=2
  E1 : Inport  Port=3
  MR1 : Inport  Port=4
  T1 : Inport  Port=5
  EB1 : Inport  Port=6
  Control : Subsystem
  Memory : Memory
  TankModel : Subsystem
  LL1 : Outport
  wires:
  TankModel/1(LiquidLevel) -> Memory/1, LL1/1
  Control/2(LiquidOut) -> TankModel/2(LiquidOut)
  Memory/1 -> Control/8(LiquidLevel)
  MR1/1 -> Control/3(ManualReference)
  CT1/1 -> Control/2(StartMaintenance), Control/1(ControlType)
  F1/1 -> Control/4(Fill)
  E1/1 -> Control/5(Empty)
  EB1/1 -> Control/6(EmergencyButton)
  T1/1 -> Control/7(Temperature)
  Control/1(LiquidIn) -> TankModel/1(LiquidIn)

== system c00007M_harness/M080/Tank1 ==
  CT1 : Inport
  F1 : Inport  Port=2
  E1 : Inport  Port=3
  MR1 : Inport  Port=4
  T1 : Inport  Port=5
  EB1 : Inport  Port=6
  Control : Subsystem
  Memory : Memory
  TankModel : Subsystem
  LL1 : Outport
  wires:
  TankModel/1(LiquidLevel) -> Memory/1, LL1/1
  Control/2(LiquidOut) -> TankModel/2(LiquidOut)
  Memory/1 -> Control/8(LiquidLevel)
  MR1/1 -> Control/3(ManualReference)
  CT1/1 -> Control/2(StartMaintenance), Control/1(ControlType)
  F1/1 -> Control/4(Fill)
  E1/1 -> Control/5(Empty)
  EB1/1 -> Control/6(EmergencyButton)
  T1/1 -> Control/7(Temperature)
  Control/1(LiquidIn) -> TankModel/1(LiquidIn)

== system c00007M_harness/M081/Tank1 ==
  CT1 : Inport
  F1 : Inport  Port=2
  E1 : Inport  Port=3
  MR1 : Inport  Port=4
  T1 : Inport  Port=5
  EB1 : Inport  Port=6
  Control : Subsystem
  Memory : Memory
  TankModel : Subsystem
  LL1 : Outport
  wires:
  TankModel/1(LiquidLevel) -> Memory/1, LL1/1
  Control/2(LiquidOut) -> TankModel/2(LiquidOut)
  Memory/1 -> Control/8(LiquidLevel)
  MR1/1 -> Control/3(ManualReference)
  CT1/1 -> Control/2(StartMaintenance), Control/1(ControlType)
  F1/1 -> Control/4(Fill)
  E1/1 -> Control/5(Empty)
  EB1/1 -> Control/6(EmergencyButton)
  T1/1 -> Control/7(Temperature)
  Control/1(LiquidIn) -> TankModel/1(LiquidIn)

== system c00007M_harness/M082/Tank1 ==
  CT1 : Inport
  F1 : Inport  Port=2
  E1 : Inport  Port=3
  MR1 : Inport  Port=4
  T1 : Inport  Port=5
  EB1 : Inport  Port=6
  Control : Subsystem
  Memory : Memory
  TankModel : Subsystem
  LL1 : Outport
  wires:
  TankModel/1(LiquidLevel) -> Memory/1, LL1/1
  Control/2(LiquidOut) -> TankModel/2(LiquidOut)
  Memory/1 -> Control/8(LiquidLevel)
  MR1/1 -> Control/3(ManualReference)
  CT1/1 -> Control/2(StartMaintenance), Control/1(ControlType)
  F1/1 -> Control/4(Fill)
  E1/1 -> Control/5(Empty)
  EB1/1 -> Control/6(EmergencyButton)
  T1/1 -> Control/7(Temperature)
  Control/1(LiquidIn) -> TankModel/1(LiquidIn)

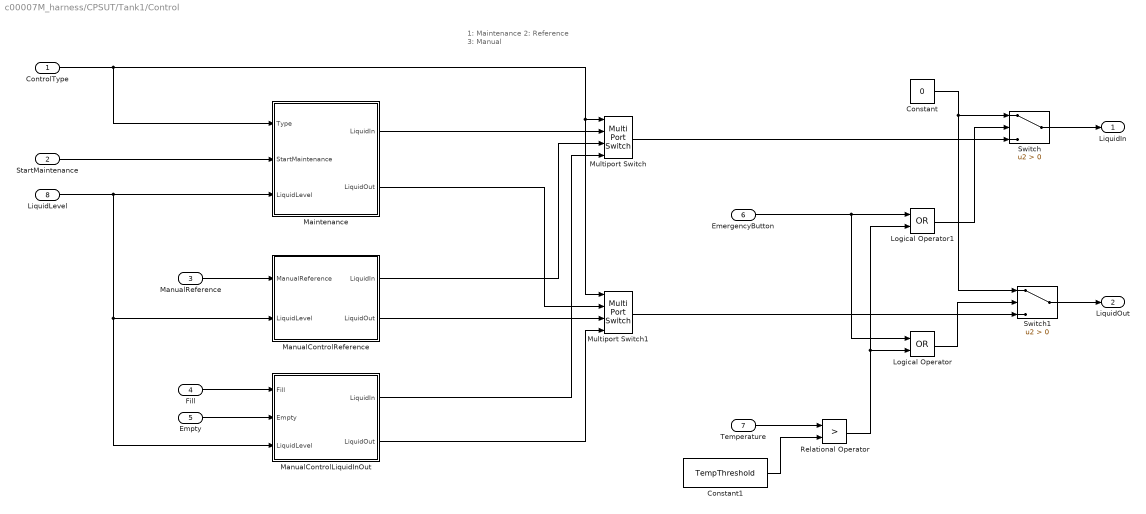
== system c00007M_harness/CPSUT/Tank1/Control ==
  note: 1: Maintenance
      | 2: Reference
      | 3: Manual
  ControlType : Inport
  StartMaintenance : Inport  Port=2
  ManualReference : Inport  Port=3
  Fill : Inport  Port=4
  Empty : Inport  Port=5
  EmergencyButton : Inport  Port=6
  Temperature : Inport  Port=7
  LiquidLevel : Inport  Port=8
  Constant : Constant  Value=0
  Constant1 : Constant  Value=TempThreshold
  Logical Operator : Logic  Operator=OR  AllPortsSameDT=off  OutDataTypeStr=boolean
  Logical Operator1 : Logic  Operator=OR  AllPortsSameDT=off  OutDataTypeStr=boolean
  Maintenance : Subsystem
  ManualControlLiquidInOut : Subsystem
  ManualControlReference : Subsystem
  Multiport Switch : MultiPortSwitch
  Multiport Switch1 : MultiPortSwitch
  Relational Operator : RelationalOperator  Operator=>  OutDataTypeStr=boolean  RndMeth=Simplest
  Switch : Switch  Criteria=u2 > Threshold
  Switch1 : Switch  Criteria=u2 > Threshold
  LiquidIn : Outport
  LiquidOut : Outport  Port=2
  wires:
  Multiport Switch/1 -> Switch/3
  Multiport Switch1/1 -> Switch1/3
  ControlType/1 -> Multiport Switch1/1, Multiport Switch/1, Maintenance/1(Type)
  Maintenance/1(LiquidIn) -> Multiport Switch/2
  ManualControlReference/1(LiquidIn) -> Multiport Switch/3
  Maintenance/2(LiquidOut) -> Multiport Switch1/2
  ManualControlReference/2(LiquidOut) -> Multiport Switch1/3
  ManualReference/1 -> ManualControlReference/1(ManualReference)
  LiquidLevel/1 -> ManualControlLiquidInOut/3(LiquidLevel), ManualControlReference/2(LiquidLevel), Maintenance/3(LiquidLevel)
  ManualControlLiquidInOut/1(LiquidIn) -> Multiport Switch/4
  ManualControlLiquidInOut/2(LiquidOut) -> Multiport Switch1/4
  Empty/1 -> ManualControlLiquidInOut/2(Empty)
  Fill/1 -> ManualControlLiquidInOut/1(Fill)
  StartMaintenance/1 -> Maintenance/2(StartMaintenance)
  Switch/1 -> LiquidIn/1
  Switch1/1 -> LiquidOut/1
  Constant/1 -> Switch1/1, Switch/1
  EmergencyButton/1 -> Logical Operator/1, Logical Operator1/1
  Relational Operator/1 -> Logical Operator1/2, Logical Operator/2
  Logical Operator/1 -> Switch1/2
  Logical Operator1/1 -> Switch/2
  Temperature/1 -> Relational Operator/1
  Constant1/1 -> Relational Operator/2

== system c00007M_harness/CPSUT/Tank1/TankModel ==
  LiquidIn : Inport
  LiquidOut : Inport  Port=2
  Add1 : Sum  Inputs=+-
  Constant1 : Constant  Value=0
  Constant2 : Constant  Value=0
  Constant3 : Constant
  Gain : Gain  Gain=1/R1
  Gain1 : Gain  Gain=1/A1
  Gain2 : Gain  Gain=1/R2
  Integrator : Integrator
  Saturation : Saturate  UpperLimit=hmax  LowerLimit=0
  Switch : Switch  Criteria=u2 ~= 0
  Switch1 : Switch  Criteria=u2 ~= 0
  LiquidLevel : Outport
  wires:
  Saturation/1 -> LiquidLevel/1, Gain2/1
  LiquidOut/1 -> Switch/2
  Add1/1 -> Gain1/1
  Gain2/1 -> Switch/1
  LiquidIn/1 -> Switch1/2
  Switch/1 -> Add1/2
  Switch1/1 -> Gain/1
  Constant2/1 -> Switch/3
  Constant3/1 -> Switch1/1
  Integrator/1 -> Saturation/1
  Gain1/1 -> Integrator/1
  Gain/1 -> Add1/1
  Constant1/1 -> Switch1/3

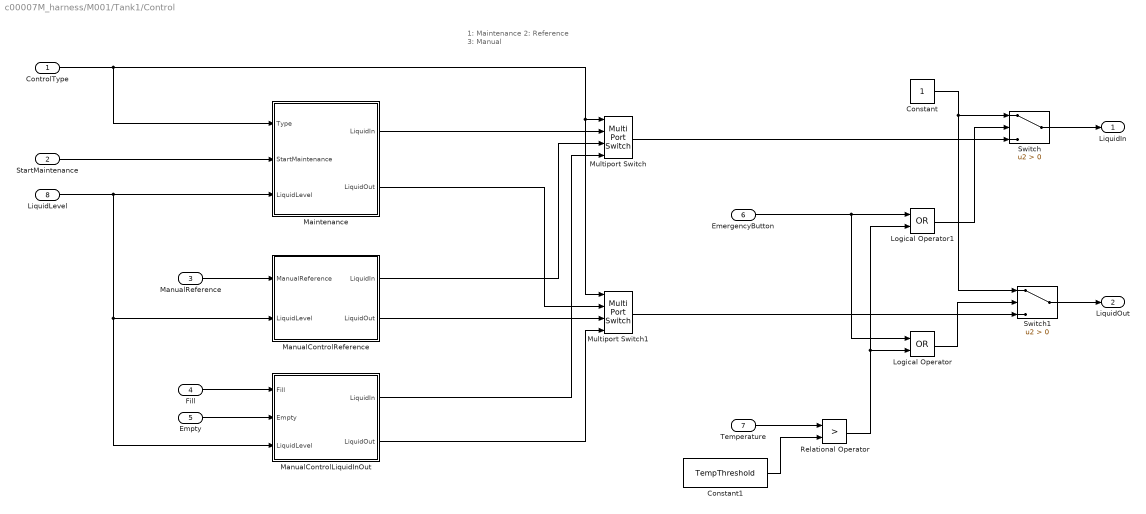
== system c00007M_harness/M001/Tank1/Control ==
  note: 1: Maintenance
      | 2: Reference
      | 3: Manual
  ControlType : Inport
  StartMaintenance : Inport  Port=2
  ManualReference : Inport  Port=3
  Fill : Inport  Port=4
  Empty : Inport  Port=5
  EmergencyButton : Inport  Port=6
  Temperature : Inport  Port=7
  LiquidLevel : Inport  Port=8
  Constant : Constant
  Constant1 : Constant  Value=TempThreshold
  Logical Operator : Logic  Operator=OR  AllPortsSameDT=off  OutDataTypeStr=boolean
  Logical Operator1 : Logic  Operator=OR  AllPortsSameDT=off  OutDataTypeStr=boolean
  Maintenance : Subsystem
  ManualControlLiquidInOut : Subsystem
  ManualControlReference : Subsystem
  Multiport Switch : MultiPortSwitch
  Multiport Switch1 : MultiPortSwitch
  Relational Operator : RelationalOperator  Operator=>  OutDataTypeStr=boolean  RndMeth=Simplest
  Switch : Switch  Criteria=u2 > Threshold
  Switch1 : Switch  Criteria=u2 > Threshold
  LiquidIn : Outport
  LiquidOut : Outport  Port=2
  wires:
  Constant1/1 -> Relational Operator/2
  Temperature/1 -> Relational Operator/1
  Logical Operator1/1 -> Switch/2
  Logical Operator/1 -> Switch1/2
  Relational Operator/1 -> Logical Operator/2, Logical Operator1/2
  EmergencyButton/1 -> Logical Operator1/1, Logical Operator/1
  Constant/1 -> Switch/1, Switch1/1
  Switch1/1 -> LiquidOut/1
  Switch/1 -> LiquidIn/1
  StartMaintenance/1 -> Maintenance/2(StartMaintenance)
  Fill/1 -> ManualControlLiquidInOut/1(Fill)
  Empty/1 -> ManualControlLiquidInOut/2(Empty)
  ManualControlLiquidInOut/2(LiquidOut) -> Multiport Switch1/4
  ManualControlLiquidInOut/1(LiquidIn) -> Multiport Switch/4
  LiquidLevel/1 -> Maintenance/3(LiquidLevel), ManualControlReference/2(LiquidLevel), ManualControlLiquidInOut/3(LiquidLevel)
  ManualReference/1 -> ManualControlReference/1(ManualReference)
  ManualControlReference/2(LiquidOut) -> Multiport Switch1/3
  Maintenance/2(LiquidOut) -> Multiport Switch1/2
  ManualControlReference/1(LiquidIn) -> Multiport Switch/3
  Maintenance/1(LiquidIn) -> Multiport Switch/2
  ControlType/1 -> Maintenance/1(Type), Multiport Switch/1, Multiport Switch1/1
  Multiport Switch1/1 -> Switch1/3
  Multiport Switch/1 -> Switch/3

== system c00007M_harness/M001/Tank1/TankModel ==
  LiquidIn : Inport
  LiquidOut : Inport  Port=2
  Add1 : Sum  Inputs=+-
  Constant1 : Constant  Value=0
  Constant2 : Constant  Value=0
  Constant3 : Constant
  Gain : Gain  Gain=1/R1
  Gain1 : Gain  Gain=1/A1
  Gain2 : Gain  Gain=1/R2
  Integrator : Integrator
  Saturation : Saturate  UpperLimit=hmax  LowerLimit=0
  Switch : Switch  Criteria=u2 ~= 0
  Switch1 : Switch  Criteria=u2 ~= 0
  LiquidLevel : Outport
  wires:
  Constant1/1 -> Switch1/3
  Gain/1 -> Add1/1
  Gain1/1 -> Integrator/1
  Integrator/1 -> Saturation/1
  Constant3/1 -> Switch1/1
  Constant2/1 -> Switch/3
  Switch1/1 -> Gain/1
  Switch/1 -> Add1/2
  LiquidIn/1 -> Switch1/2
  Gain2/1 -> Switch/1
  Add1/1 -> Gain1/1
  LiquidOut/1 -> Switch/2
  Saturation/1 -> Gain2/1, LiquidLevel/1

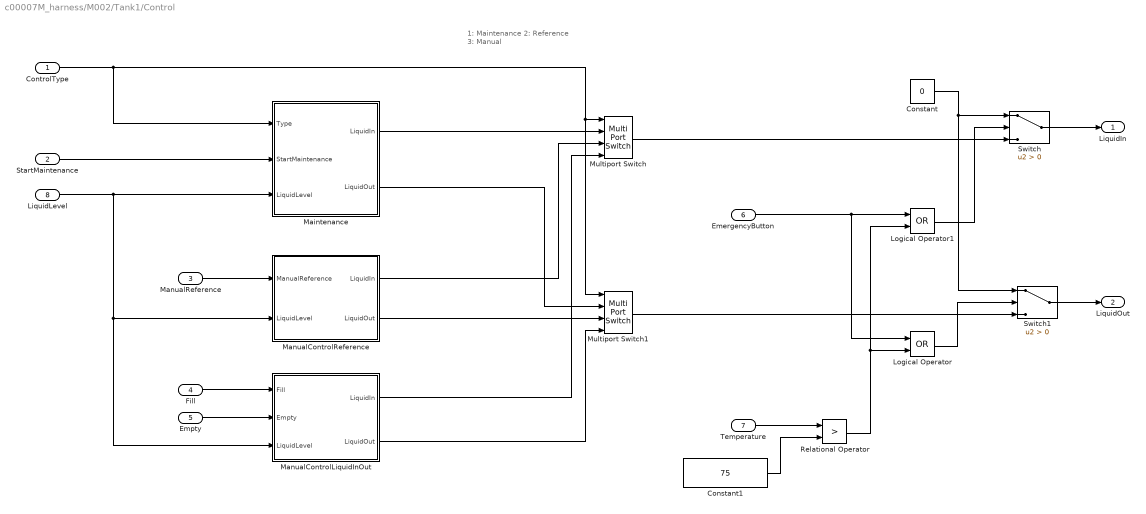
== system c00007M_harness/M002/Tank1/Control ==
  note: 1: Maintenance
      | 2: Reference
      | 3: Manual
  ControlType : Inport
  StartMaintenance : Inport  Port=2
  ManualReference : Inport  Port=3
  Fill : Inport  Port=4
  Empty : Inport  Port=5
  EmergencyButton : Inport  Port=6
  Temperature : Inport  Port=7
  LiquidLevel : Inport  Port=8
  Constant : Constant  Value=0
  Constant1 : Constant  Value=75
  Logical Operator : Logic  Operator=OR  AllPortsSameDT=off  OutDataTypeStr=boolean
  Logical Operator1 : Logic  Operator=OR  AllPortsSameDT=off  OutDataTypeStr=boolean
  Maintenance : Subsystem
  ManualControlLiquidInOut : Subsystem
  ManualControlReference : Subsystem
  Multiport Switch : MultiPortSwitch
  Multiport Switch1 : MultiPortSwitch
  Relational Operator : RelationalOperator  Operator=>  OutDataTypeStr=boolean  RndMeth=Simplest
  Switch : Switch  Criteria=u2 > Threshold
  Switch1 : Switch  Criteria=u2 > Threshold
  LiquidIn : Outport
  LiquidOut : Outport  Port=2
  wires:
  Multiport Switch/1 -> Switch/3
  Multiport Switch1/1 -> Switch1/3
  ControlType/1 -> Multiport Switch1/1, Multiport Switch/1, Maintenance/1(Type)
  Maintenance/1(LiquidIn) -> Multiport Switch/2
  ManualControlReference/1(LiquidIn) -> Multiport Switch/3
  Maintenance/2(LiquidOut) -> Multiport Switch1/2
  ManualControlReference/2(LiquidOut) -> Multiport Switch1/3
  ManualReference/1 -> ManualControlReference/1(ManualReference)
  LiquidLevel/1 -> ManualControlLiquidInOut/3(LiquidLevel), ManualControlReference/2(LiquidLevel), Maintenance/3(LiquidLevel)
  ManualControlLiquidInOut/1(LiquidIn) -> Multiport Switch/4
  ManualControlLiquidInOut/2(LiquidOut) -> Multiport Switch1/4
  Empty/1 -> ManualControlLiquidInOut/2(Empty)
  Fill/1 -> ManualControlLiquidInOut/1(Fill)
  StartMaintenance/1 -> Maintenance/2(StartMaintenance)
  Switch/1 -> LiquidIn/1
  Switch1/1 -> LiquidOut/1
  Constant/1 -> Switch1/1, Switch/1
  EmergencyButton/1 -> Logical Operator/1, Logical Operator1/1
  Relational Operator/1 -> Logical Operator1/2, Logical Operator/2
  Logical Operator/1 -> Switch1/2
  Logical Operator1/1 -> Switch/2
  Temperature/1 -> Relational Operator/1
  Constant1/1 -> Relational Operator/2
